simulink model "Model"  (R2015b)
settings: Solver=ode4  StartTime=0.0  StopTime=15  FixedStep=0.015  RelTol=1e-3
undefined symbols (not defined in the file or in its folder): Earth, WGS84
libraries: aerolibutil x3, aerolibfltsims x2, aerolibtransform2 x1
settings Model: Creator=A7med Al-Dakrory  LastModifiedBy=Ahmed
settings DataIOCC: SaveFormat=Array
settings DebuggingCC: AllowSymbolicDim=on
settings HardwareCC: ProdBitPerPointer=32  ProdLargestAtomicFloat=None  ProdIntDivRoundTo=Undefined  ProdEndianess=Unspecified  ProdWordSize=32  ProdHWDeviceType=32-bit Generic
settings GRTTargetCC: GeneratePreprocessorConditionals=Disable all
settings ConfigComp: CovModelRefEnable=Off

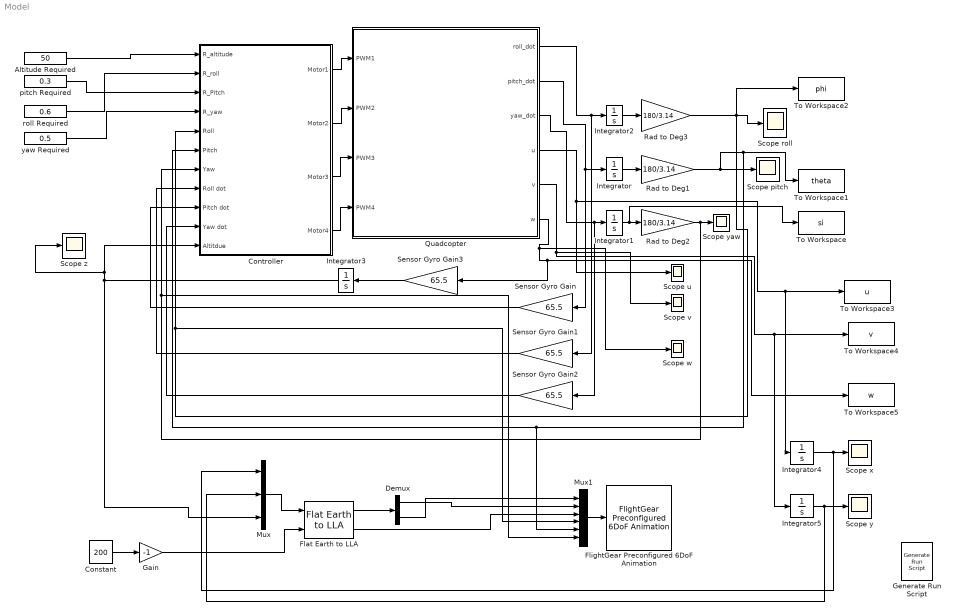
== system Model ==
  Altitude Required : Constant  Value=50
  Constant : Constant  Value=200
  Controller : Subsystem
  Demux : Demux  Outputs=2
  Flat Earth to LLA : aerolibtransform2/Flat Earth to LLA  units=Metric (MKS)  ptype=Earth (WGS84)  F=1/298.257223563  R=6378137  LL0=[34.9100 -117.8912]  psi=0
  FlightGear Preconfigured 6DoF Animation : aerolibfltsims/FlightGear Preconfigured 6DoF Animation  xFlightGearVersion=v3.0  DestinationIpAddress=127.0.0.1  DestinationPort=5502  SampleTime=15/1000
  Gain : Gain  Gain=-1
  Generate Run Script : aerolibfltsims/Generate Run Script  OutputFileName=runfg.bat  FlightGearBaseDirectory=C:\Program Files\FlightGear  GeometryModelName=HL20  DestinationPort=5502  OriginAddress=127.0.0.1  OriginPort=5505  LocalAddress=127.0.0.1  AirportId=KSFO  RunwayId=10L  InitialAltitude=200  InitialHeading=0  OffsetDistance=0  OffsetAzimuth=0  GenerateFile=off  Architecture=Default  dataFlow=Send
  Integrator{,1..5} (6 alike) : Integrator
  Mux : Mux  Inputs=3
  Mux1 : Mux  Inputs=6
  Quadcopter : Subsystem
      mask Display:
      | port_label('output', 1, 'roll_dot')
      | port_label('output', 2, 'pitch_dot')
      | port_label('output', 3, 'yaw_dot')
      | port_label('output', 4, 'u')
      | port_label('output', 5, 'v')
      | port_label('output', 6, 'w')
      | port_label('input', 1, 'Motor1')
      | port_label('input', 2, 'Motor2')
      | port_label('input', 3, 'Motor3')
      | port_label('input', 4, 'Motor4')
  Rad to Deg1 : Gain  Gain=180/3.14
  Rad to Deg2 : Gain  Gain=180/3.14
  Rad to Deg3 : Gain  Gain=180/3.14
  Scope pitch : Scope
  Scope roll : Scope
  Scope u : Scope
  Scope v : Scope
  Scope w : Scope
  Scope x : Scope
  "Scope y " : Scope
  Scope yaw : Scope
  Scope z : Scope
  Sensor Gyro Gain{,1..3} (4 alike) : Gain  Gain=65.5
  To Workspace : ToWorkspace  VariableName=si  SaveFormat=Timeseries  SampleTime=-1
  To Workspace1 : ToWorkspace  VariableName=theta  SaveFormat=Timeseries  SampleTime=-1
  To Workspace2 : ToWorkspace  VariableName=phi  SaveFormat=Timeseries  SampleTime=-1
  To Workspace3 : ToWorkspace  VariableName=u  SaveFormat=Timeseries  SampleTime=-1
  To Workspace4 : ToWorkspace  VariableName=v  SaveFormat=Timeseries  SampleTime=-1
  To Workspace5 : ToWorkspace  VariableName=w  SaveFormat=Timeseries  SampleTime=-1
  pitch Required : Constant  Value=0.3
  roll Required : Constant  Value=0.6
  yaw Required : Constant  Value=0.5
  wires:
  Rad to Deg1/1 -> Mux1/5, Controller/6(Pitch), To Workspace1/1, Scope pitch/1
  Integrator/1 -> Rad to Deg1/1
  Quadcopter/2(pitch_dot) -> Sensor Gyro Gain/1, Integrator/1
  Integrator1/1 -> To Workspace/1, Rad to Deg2/1
  Quadcopter/3(yaw_dot) -> Sensor Gyro Gain2/1, Integrator1/1
  Rad to Deg2/1 -> Controller/7(Yaw), Mux1/6, Scope yaw/1
  Integrator2/1 -> Rad to Deg3/1
  Quadcopter/1(roll_dot) -> Sensor Gyro Gain1/1, Integrator2/1
  Quadcopter/4(u) -> Integrator4/1, To Workspace3/1, Scope u/1
  Quadcopter/5(v) -> Integrator5/1, To Workspace4/1, Scope v/1
  Quadcopter/6(w) -> Sensor Gyro Gain3/1, To Workspace5/1, Scope w/1
  Controller/4(Motor4) -> Quadcopter/4(PWM4)
  Rad to Deg3/1 -> Scope roll/1, To Workspace2/1, Controller/5(Roll), Mux1/4
  Integrator3/1 -> Controller/11(Altitdue), Scope z/1, Mux/3
  Controller/3(Motor3) -> Quadcopter/3(PWM3)
  Controller/2(Motor2) -> Quadcopter/2(PWM2)
  Controller/1(Motor1) -> Quadcopter/1(PWM1)
  Altitude Required/1 -> Controller/1(R_altitude)
  yaw Required/1 -> Controller/4(R_yaw)
  pitch Required/1 -> Controller/3(R_Pitch)
  roll Required/1 -> Controller/2(R_roll)
  Sensor Gyro Gain2/1 -> Controller/10(Yaw dot)
  Sensor Gyro Gain/1 -> Controller/9(Pitch dot)
  Sensor Gyro Gain1/1 -> Controller/8(Roll dot)
  Sensor Gyro Gain3/1 -> Integrator3/1
  Mux/1 -> Flat Earth to LLA/1
  Integrator5/1 -> Mux/2, "Scope y "/1
  Integrator4/1 -> Mux/1, Scope x/1
  Flat Earth to LLA/1 -> Demux/1
  Mux1/1 -> FlightGear Preconfigured 6DoF Animation/1
  Flat Earth to LLA/2 -> Mux1/3
  Gain/1 -> Flat Earth to LLA/2
  Demux/1 -> Mux1/2
  Demux/2 -> Mux1/1
  Constant/1 -> Gain/1

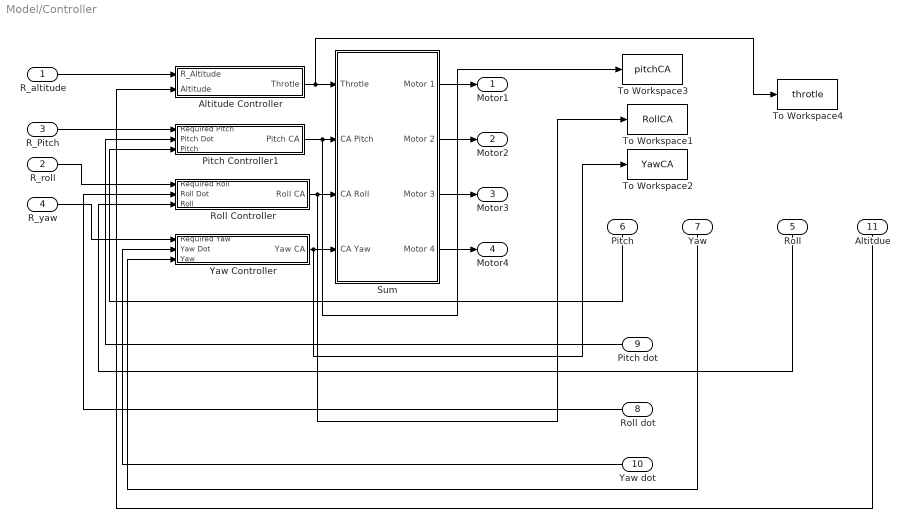
== system Model/Controller ==
  R_altitude : Inport
  R_roll : Inport  Port=2
  R_Pitch : Inport  Port=3
  R_yaw : Inport  Port=4
  Roll : Inport  Port=5
  Pitch : Inport  Port=6
  Yaw : Inport  Port=7
  Roll dot : Inport  Port=8
  Pitch dot : Inport  Port=9
  Yaw dot : Inport  Port=10
  Altitdue : Inport  Port=11
  Altitude Controller : Subsystem
  Pitch Controller1 : Subsystem
  Roll Controller : Subsystem
  Sum : Subsystem
  To Workspace1 : ToWorkspace  VariableName=RollCA  SaveFormat=Timeseries  SampleTime=-1
  To Workspace2 : ToWorkspace  VariableName=YawCA  SaveFormat=Timeseries  SampleTime=-1
  To Workspace3 : ToWorkspace  VariableName=pitchCA  SaveFormat=Timeseries  SampleTime=-1
  To Workspace4 : ToWorkspace  VariableName=throtle  SaveFormat=Timeseries  SampleTime=-1
  Yaw Controller : Subsystem
  Motor1 : Outport
  Motor2 : Outport  Port=2
  Motor3 : Outport  Port=3
  Motor4 : Outport  Port=4
  wires:
  Pitch Controller1/1(Pitch CA) -> To Workspace3/1, Sum/2(CA Pitch)
  Pitch dot/1 -> Pitch Controller1/2(Pitch Dot)
  R_Pitch/1 -> Pitch Controller1/1(Required Pitch)
  Sum/1(Motor 1) -> Motor1/1
  Sum/2(Motor 2) -> Motor2/1
  Sum/3(Motor 3) -> Motor3/1
  Sum/4(Motor 4) -> Motor4/1
  Roll dot/1 -> Roll Controller/2(Roll Dot)
  Yaw/1 -> Yaw Controller/3(Yaw)
  Roll/1 -> Roll Controller/3(Roll)
  Pitch/1 -> Pitch Controller1/3(Pitch)
  Yaw dot/1 -> Yaw Controller/2(Yaw Dot)
  Roll Controller/1(Roll CA) -> To Workspace1/1, Sum/3(CA Roll)
  Yaw Controller/1(Yaw CA) -> To Workspace2/1, Sum/4(CA Yaw)
  R_roll/1 -> Roll Controller/1(Required Roll)
  R_yaw/1 -> Yaw Controller/1(Required Yaw)
  R_altitude/1 -> Altitude Controller/1(R_Altitude)
  Altitude Controller/1(Throtle) -> To Workspace4/1, Sum/1(Throtle)
  Altitdue/1 -> Altitude Controller/2(Altitude)

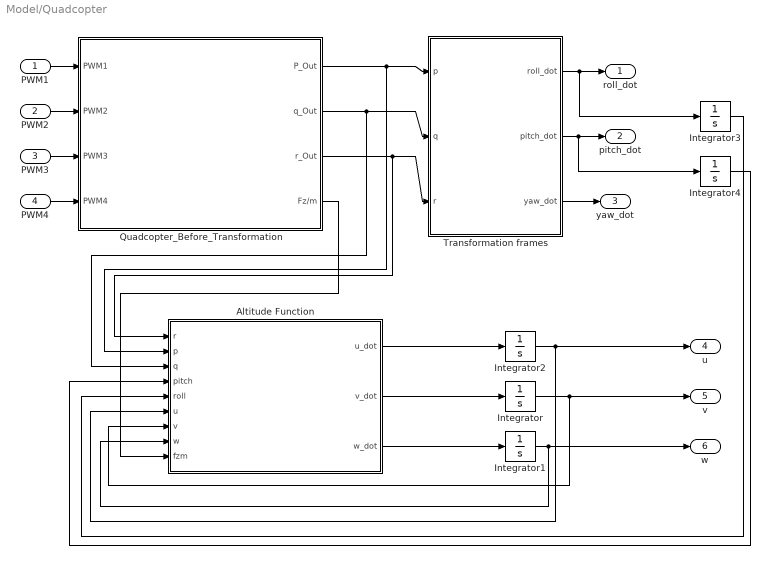
== system Model/Quadcopter ==
  PWM1 : Inport
  PWM2 : Inport  Port=2
  PWM3 : Inport  Port=3
  PWM4 : Inport  Port=4
  Altitude Function : MATLAB Function  TreatAsAtomicUnit=on
      settings: PermitHierarchicalResolution=ParametersOnly
  Integrator{,1..4} (5 alike) : Integrator
  Quadcopter_Before_Transformation : Subsystem
      mask Display:
      | port_label('output', 1, 'roll rate')
      | port_label('output', 2, 'pitch rate')
      | port_label('output', 3, 'yaw rate')
      | port_label('output', 4, 'Fz/m')
      | port_label('input', 1, 'PWM 1')
      | port_label('input', 2, 'PWM 2')
      | port_label('input', 3, 'PWM 3')
      | port_label('input', 4, 'PWM 4')
  Transformation frames : Subsystem
  roll_dot : Outport
  pitch_dot : Outport  Port=2
  yaw_dot : Outport  Port=3
  u : Outport  Port=4
  v : Outport  Port=5
  w : Outport  Port=6
  wires:
  PWM2/1 -> Quadcopter_Before_Transformation/2(PWM2)
  Quadcopter_Before_Transformation/3(r_Out) -> Altitude Function/1(r), Transformation frames/3(r)
  Quadcopter_Before_Transformation/1(P_Out) -> Altitude Function/2(p), Transformation frames/1(p)
  PWM1/1 -> Quadcopter_Before_Transformation/1(PWM1)
  Quadcopter_Before_Transformation/2(q_Out) -> Altitude Function/3(q), Transformation frames/2(q)
  Transformation frames/2(pitch_dot) -> Integrator4/1, pitch_dot/1
  Transformation frames/3(yaw_dot) -> yaw_dot/1
  Transformation frames/1(roll_dot) -> Integrator3/1, roll_dot/1
  PWM3/1 -> Quadcopter_Before_Transformation/3(PWM3)
  PWM4/1 -> Quadcopter_Before_Transformation/4(PWM4)
  Altitude Function/2(v_dot) -> Integrator/1
  Altitude Function/3(w_dot) -> Integrator1/1
  Altitude Function/1(u_dot) -> Integrator2/1
  Integrator4/1 -> Altitude Function/4(pitch)
  Integrator3/1 -> Altitude Function/5(roll)
  Integrator2/1 -> u/1, Altitude Function/6(u)
  Integrator/1 -> Altitude Function/7(v), v/1
  Integrator1/1 -> Altitude Function/8(w), w/1
  Quadcopter_Before_Transformation/4(Fz/m) -> Altitude Function/9(fzm)

== system Model/Controller/Altitude Controller ==
  R_Altitude : Inport
  Altitude : Inport  Port=2
  PID Altitude : Subsystem
  Sum : Sum  Inputs=|+-
  Throtle : Outport
  wires:
  Sum/1 -> PID Altitude/1(Error)
  R_Altitude/1 -> Sum/2
  Altitude/1 -> Sum/1
  PID Altitude/1(Output) -> Throtle/1

== system Model/Controller/Pitch Controller1 ==
  Required Pitch : Inport
  Pitch Dot : Inport  Port=2
  Pitch : Inport  Port=3
  PID Pitch : Subsystem
  PID Pitch Rate : Subsystem
  Sum2 : Sum  Inputs=|++
  Sum3 : Sum  Inputs=|+-
  Pitch CA : Outport
  wires:
  Required Pitch/1 -> Sum3/1
  Sum3/1 -> PID Pitch/1(Error)
  Pitch Dot/1 -> PID Pitch Rate/1(Error)
  Pitch/1 -> Sum3/2
  PID Pitch/1(Output) -> Sum2/1
  PID Pitch Rate/1(Output) -> Sum2/2
  Sum2/1 -> Pitch CA/1

== system Model/Controller/Roll Controller ==
  Required Roll : Inport
  Roll Dot : Inport  Port=2
  Roll : Inport  Port=3
  PID Roll : Subsystem
  PID Roll Rate : Subsystem
  Sum2 : Sum  Inputs=|++
  Sum3 : Sum  Inputs=|+-
  Roll CA : Outport
  wires:
  Required Roll/1 -> Sum3/1
  Sum3/1 -> PID Roll/1(Error)
  Roll Dot/1 -> PID Roll Rate/1(Error)
  Roll/1 -> Sum3/2
  PID Roll/1(Output) -> Sum2/1
  PID Roll Rate/1(Output) -> Sum2/2
  Sum2/1 -> Roll CA/1

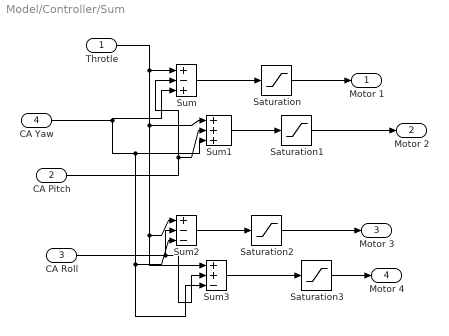
== system Model/Controller/Sum ==
  Throtle : Inport
  CA Pitch : Inport  Port=2
  CA Roll : Inport  Port=3
  CA Yaw : Inport  Port=4
  Saturation{,1..3} (4 alike) : Saturate  UpperLimit=1950  LowerLimit=1050
  Sum : Sum  Inputs=+-+
  Sum1 : Sum  Inputs=+++
  Sum2 : Sum  Inputs=+--
  Sum3 : Sum  Inputs=++-
  Motor 1 : Outport
  Motor 2 : Outport  Port=2
  Motor 3 : Outport  Port=3
  Motor 4 : Outport  Port=4
  wires:
  CA Pitch/1 -> Sum/2, Sum1/2
  Saturation/1 -> Motor 1/1
  Sum/1 -> Saturation/1
  Sum1/1 -> Saturation1/1
  Saturation1/1 -> Motor 2/1
  Throtle/1 -> Sum3/1, Sum2/1, Sum1/1, Sum/1
  CA Roll/1 -> Sum3/2, Sum2/2
  Saturation2/1 -> Motor 3/1
  Sum2/1 -> Saturation2/1
  Sum3/1 -> Saturation3/1
  Saturation3/1 -> Motor 4/1
  CA Yaw/1 -> Sum/3, Sum3/3, Sum2/3, Sum1/3

== system Model/Controller/Yaw Controller ==
  Required Yaw : Inport
  Yaw Dot : Inport  Port=2
  Yaw : Inport  Port=3
  PID Yaw : Subsystem
  PID Yaw Rate : Subsystem
  Sum2 : Sum  Inputs=|++
  Sum3 : Sum  Inputs=|+-
  Yaw CA : Outport
  wires:
  Required Yaw/1 -> Sum3/1
  Sum3/1 -> PID Yaw/1(Error)
  Yaw Dot/1 -> PID Yaw Rate/1(Error)
  Yaw/1 -> Sum3/2
  PID Yaw/1(Output) -> Sum2/1
  PID Yaw Rate/1(Output) -> Sum2/2
  Sum2/1 -> Yaw CA/1

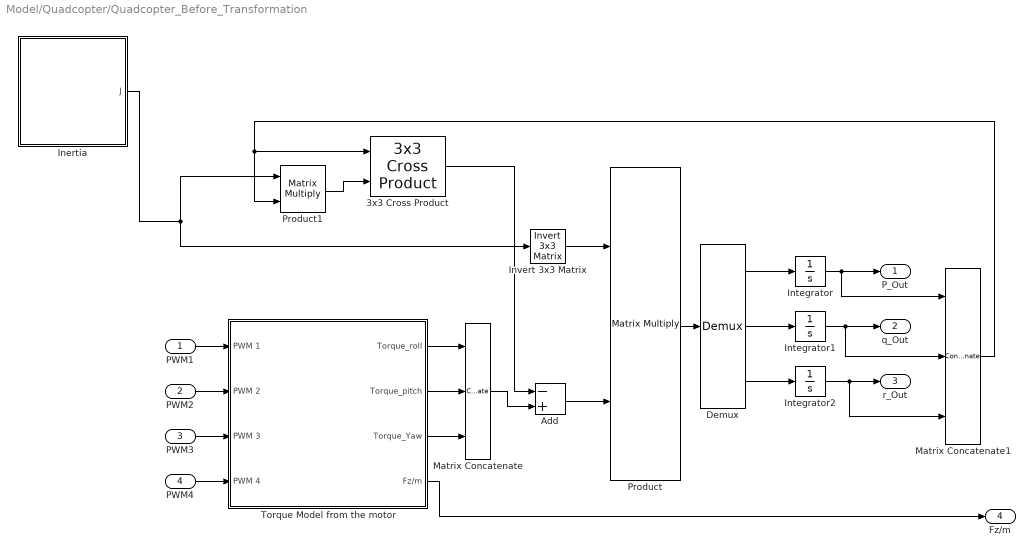
== system Model/Quadcopter/Quadcopter_Before_Transformation ==
  PWM1 : Inport
  PWM2 : Inport  Port=2
  PWM3 : Inport  Port=3
  PWM4 : Inport  Port=4
  3x3 Cross Product : aerolibutil/3x3 Cross Product
  Add : Sum  Inputs=-+
  Demux : Demux  Outputs=3
  Inertia : Subsystem
  Integrator : Integrator
  Integrator1 : Integrator
  Integrator2 : Integrator
  Invert 3x3 Matrix : aerolibutil/Invert  3x3 Matrix
  Matrix Concatenate : Concatenate  NumInputs=3  ConcatenateDimension=2
  Matrix Concatenate1 : Concatenate  NumInputs=3  ConcatenateDimension=2
  Product : Product  Multiplication=Matrix(*)
  Product1 : Product  Multiplication=Matrix(*)
  Torque Model from the motor : Subsystem
      mask Display:
      | port_label('output', 1, 'Torque_Roll')
      | port_label('output', 2, 'Torque_pitch')
      | port_label('output', 3, 'Torque_yaw')
      | port_label('output', 4, 'Fz/m')
      | port_label('input', 1, 'PWM 1')
      | port_label('input', 2, 'PWM 2')
      | port_label('input', 3, 'PWM 3')
      | port_label('input', 4, 'PWM 4')
  P_Out : Outport
  q_Out : Outport  Port=2
  r_Out : Outport  Port=3
  Fz/m : Outport  Port=4
  wires:
  Demux/1 -> Integrator/1
  Torque Model from the motor/1("Torque_roll ") -> Matrix Concatenate/1
  Product/1 -> Demux/1
  Integrator2/1 -> Matrix Concatenate1/3, r_Out/1
  Integrator/1 -> Matrix Concatenate1/1, P_Out/1
  Integrator1/1 -> Matrix Concatenate1/2, q_Out/1
  PWM2/1 -> Torque Model from the motor/2(PWM 2)
  PWM4/1 -> Torque Model from the motor/4(PWM 4)
  PWM3/1 -> Torque Model from the motor/3(PWM 3)
  PWM1/1 -> Torque Model from the motor/1(PWM 1)
  Invert 3x3 Matrix/1 -> Product/1
  Demux/3 -> Integrator2/1
  Demux/2 -> Integrator1/1
  Torque Model from the motor/2(Torque_pitch) -> Matrix Concatenate/2
  Torque Model from the motor/3("Torque_Yaw ") -> Matrix Concatenate/3
  Matrix Concatenate/1 -> Add/2
  Add/1 -> Product/2
  Matrix Concatenate1/1 -> Product1/2, 3x3 Cross Product/1
  Inertia/1(J) -> Invert 3x3 Matrix/1, Product1/1
  Product1/1 -> 3x3 Cross Product/2
  3x3 Cross Product/1 -> Add/1
  Torque Model from the motor/4(Fz/m) -> Fz/m/1

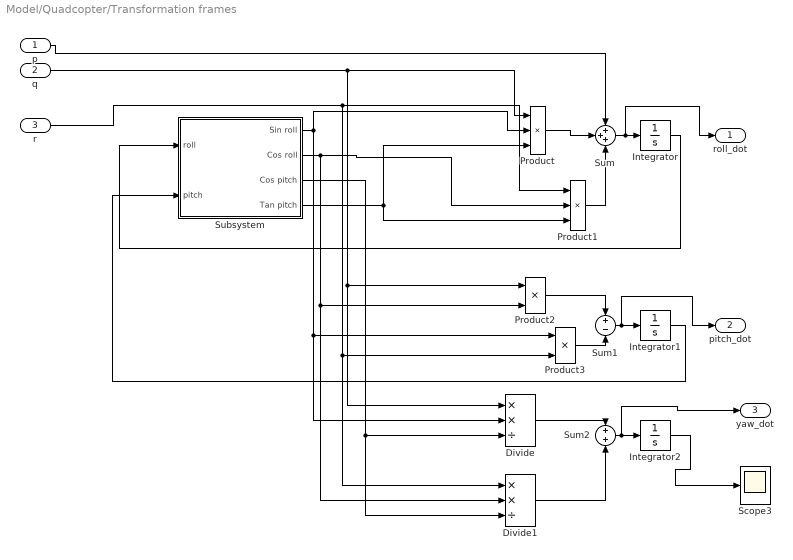
== system Model/Quadcopter/Transformation frames ==
  p : Inport
  q : Inport  Port=2
  r : Inport  Port=3
  Divide : Product  Inputs=**/
  Divide1 : Product  Inputs=**/
  Integrator : Integrator
  Integrator1 : Integrator
  Integrator2 : Integrator
  Product : Product  Inputs=3
  Product1 : Product  Inputs=3
  Product2 : Product
  Product3 : Product
  Scope3 : Scope
  Subsystem : Subsystem
  Sum : Sum  Inputs=+++
  Sum1 : Sum  Inputs=+-
  Sum2 : Sum
  roll_dot : Outport
  pitch_dot : Outport  Port=2
  yaw_dot : Outport  Port=3
  wires:
  Integrator/1 -> Subsystem/1(roll)
  p/1 -> Sum/1
  Subsystem/2(Cos roll) -> Divide1/2, Product2/2, Product1/2
  Sum/1 -> roll_dot/1, Integrator/1
  Subsystem/4(Tan pitch) -> Product1/3, Product/3
  q/1 -> Divide/1, Product2/1, Product/1
  r/1 -> Divide1/1, Product3/2, Product1/1
  Sum2/1 -> yaw_dot/1, Integrator2/1
  Sum1/1 -> pitch_dot/1, Integrator1/1
  Integrator1/1 -> Subsystem/2(pitch)
  Subsystem/1(Sin roll) -> Divide/2, Product3/1, Product/2
  Integrator2/1 -> Scope3/1
  Product/1 -> Sum/2
  Product1/1 -> Sum/3
  Product2/1 -> Sum1/1
  Product3/1 -> Sum1/2
  Divide/1 -> Sum2/1
  Subsystem/3(Cos pitch) -> Divide1/3, Divide/3
  Divide1/1 -> Sum2/2

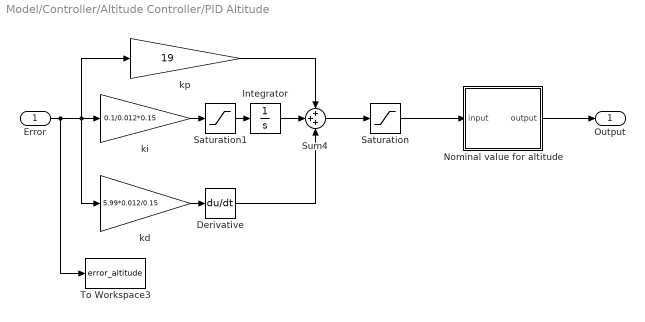
== system Model/Controller/Altitude Controller/PID Altitude ==
  Error : Inport
  Derivative : Derivative
  Integrator : Integrator
  Nominal value for altitude : MATLAB Function  TreatAsAtomicUnit=on
      settings: PermitHierarchicalResolution=ParametersOnly
  Saturation : Saturate  UpperLimit=20  LowerLimit=0
  Saturation1 : Saturate  UpperLimit=20  LowerLimit=-20
  Sum4 : Sum  Inputs=+++
  To Workspace3 : ToWorkspace  VariableName=error_altitude  SaveFormat=Timeseries  SampleTime=-1
  kd : Gain  Gain=5.99*0.012/0.15
  ki : Gain  Gain=0.1/0.012*0.15
  kp : Gain  Gain=19
  Output : Outport
  wires:
  Integrator/1 -> Sum4/2
  kd/1 -> Derivative/1
  Error/1 -> To Workspace3/1, kd/1, ki/1, kp/1
  kp/1 -> Sum4/1
  Derivative/1 -> Sum4/3
  Sum4/1 -> Saturation/1
  Saturation/1 -> Nominal value for altitude/1(input)
  Nominal value for altitude/1(output) -> Output/1
  ki/1 -> Saturation1/1
  Saturation1/1 -> Integrator/1

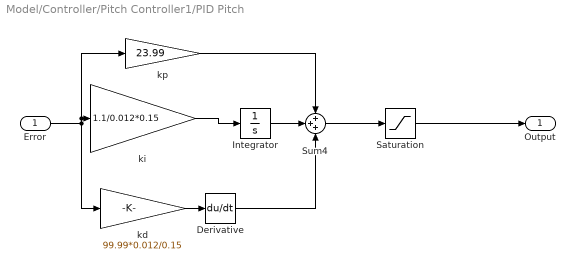
== system Model/Controller/Pitch Controller1/PID Pitch ==
  Error : Inport
  Derivative : Derivative
  Integrator : Integrator
  Saturation : Saturate  UpperLimit=150  LowerLimit=-150
  Sum4 : Sum  Inputs=+++
  kd : Gain  Gain=99.99*0.012/0.15
  ki : Gain  Gain=1.1/0.012*0.15
  kp : Gain  Gain=23.99
  Output : Outport
  wires:
  Integrator/1 -> Sum4/2
  kd/1 -> Derivative/1
  Error/1 -> ki/1, kp/1, kd/1
  kp/1 -> Sum4/1
  Derivative/1 -> Sum4/3
  ki/1 -> Integrator/1
  Saturation/1 -> Output/1
  Sum4/1 -> Saturation/1

== system Model/Controller/Pitch Controller1/PID Pitch Rate ==
  Error : Inport
  Derivative : Derivative
  Integrator : Integrator
  Sum4 : Sum  Inputs=+++
  kd : Gain  Gain=-89.99*0.01*0.012/0.15
  ki : Gain  Gain=0
  kp : Gain  Gain=-0.01*23.9
  Output : Outport
  wires:
  ki/1 -> Integrator/1
  Derivative/1 -> Sum4/3
  kp/1 -> Sum4/1
  Error/1 -> kd/1, kp/1, ki/1
  kd/1 -> Derivative/1
  Integrator/1 -> Sum4/2
  Sum4/1 -> Output/1

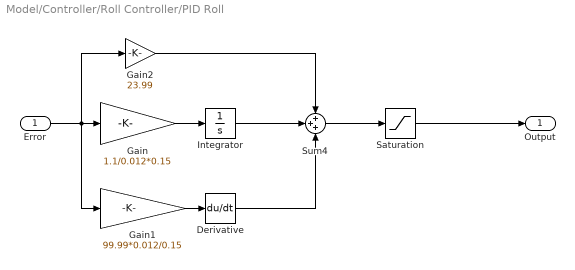
== system Model/Controller/Roll Controller/PID Roll ==
  Error : Inport
  Derivative : Derivative
  Gain : Gain  Gain=1.1/0.012*0.15
  Gain1 : Gain  Gain=99.99*0.012/0.15
  Gain2 : Gain  Gain=23.99
  Integrator : Integrator
  Saturation : Saturate  UpperLimit=150  LowerLimit=-150
  Sum4 : Sum  Inputs=+++
  Output : Outport
  wires:
  Integrator/1 -> Sum4/2
  Gain1/1 -> Derivative/1
  Error/1 -> Gain1/1, Gain/1, Gain2/1
  Gain2/1 -> Sum4/1
  Derivative/1 -> Sum4/3
  Gain/1 -> Integrator/1
  Saturation/1 -> Output/1
  Sum4/1 -> Saturation/1

== system Model/Controller/Roll Controller/PID Roll Rate ==
  Error : Inport
  Derivative : Derivative
  Gain : Gain  Gain=0
  Gain1 : Gain  Gain=-89.99*0.01*0.012/0.15
  Gain2 : Gain  Gain=-0.01*23.9
  Integrator : Integrator
  Sum4 : Sum  Inputs=+++
  Output : Outport
  wires:
  Gain/1 -> Integrator/1
  Derivative/1 -> Sum4/3
  Gain2/1 -> Sum4/1
  Error/1 -> Gain1/1, Gain2/1, Gain/1
  Gain1/1 -> Derivative/1
  Integrator/1 -> Sum4/2
  Sum4/1 -> Output/1

== system Model/Controller/Yaw Controller/PID Yaw ==
  Error : Inport
  Derivative : Derivative
  Gain : Gain  Gain=1.1/0.012*0.15
  Gain1 : Gain  Gain=99.99*0.012/0.15
  Gain2 : Gain  Gain=23.99
  Integrator : Integrator
  Saturation : Saturate  UpperLimit=150  LowerLimit=-150
  Sum4 : Sum  Inputs=+++
  Output : Outport
  wires:
  Integrator/1 -> Sum4/2
  Gain1/1 -> Derivative/1
  Error/1 -> Gain1/1, Gain/1, Gain2/1
  Gain2/1 -> Sum4/1
  Derivative/1 -> Sum4/3
  Gain/1 -> Integrator/1
  Saturation/1 -> Output/1
  Sum4/1 -> Saturation/1

== system Model/Controller/Yaw Controller/PID Yaw Rate ==
  Error : Inport
  Derivative : Derivative
  Gain : Gain  Gain=0
  Gain1 : Gain  Gain=-89.99*0.01*0.012/0.15
  Gain2 : Gain  Gain=-0.01*23.9
  Integrator : Integrator
  Sum4 : Sum  Inputs=+++
  Output : Outport
  wires:
  Gain/1 -> Integrator/1
  Derivative/1 -> Sum4/3
  Gain2/1 -> Sum4/1
  Error/1 -> Gain1/1, Gain2/1, Gain/1
  Gain1/1 -> Derivative/1
  Integrator/1 -> Sum4/2
  Sum4/1 -> Output/1

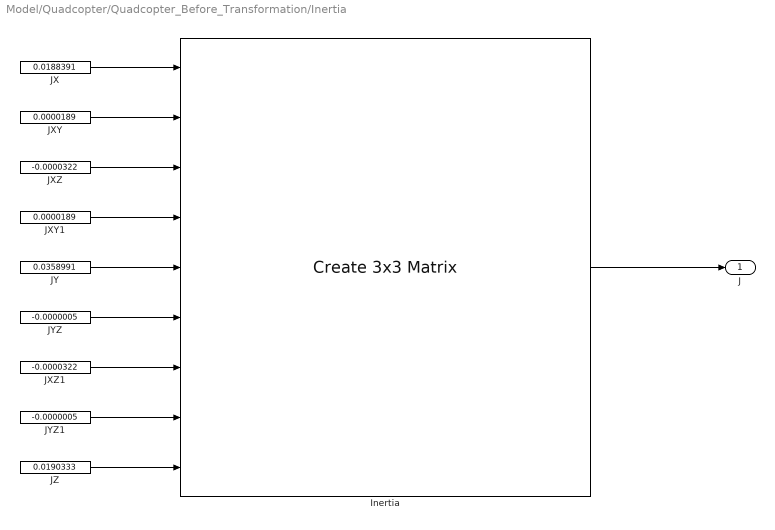
== system Model/Quadcopter/Quadcopter_Before_Transformation/Inertia ==
  Inertia : aerolibutil/Create 3x3 Matrix
  JX : Constant  Value=0.0188391
  JXY : Constant  Value=0.0000189
  JXY1 : Constant  Value=0.0000189
  JXZ : Constant  Value=-0.0000322
  JXZ1 : Constant  Value=-0.0000322
  JY : Constant  Value=0.0358991
  JYZ : Constant  Value=-0.0000005
  JYZ1 : Constant  Value=-0.0000005
  JZ : Constant  Value=0.0190333
  J : Outport
  wires:
  JYZ/1 -> Inertia/6
  JZ/1 -> Inertia/9
  JXY/1 -> Inertia/2
  JXZ/1 -> Inertia/3
  JY/1 -> Inertia/5
  JX/1 -> Inertia/1
  Inertia/1 -> J/1
  JXY1/1 -> Inertia/4
  JXZ1/1 -> Inertia/7
  JYZ1/1 -> Inertia/8

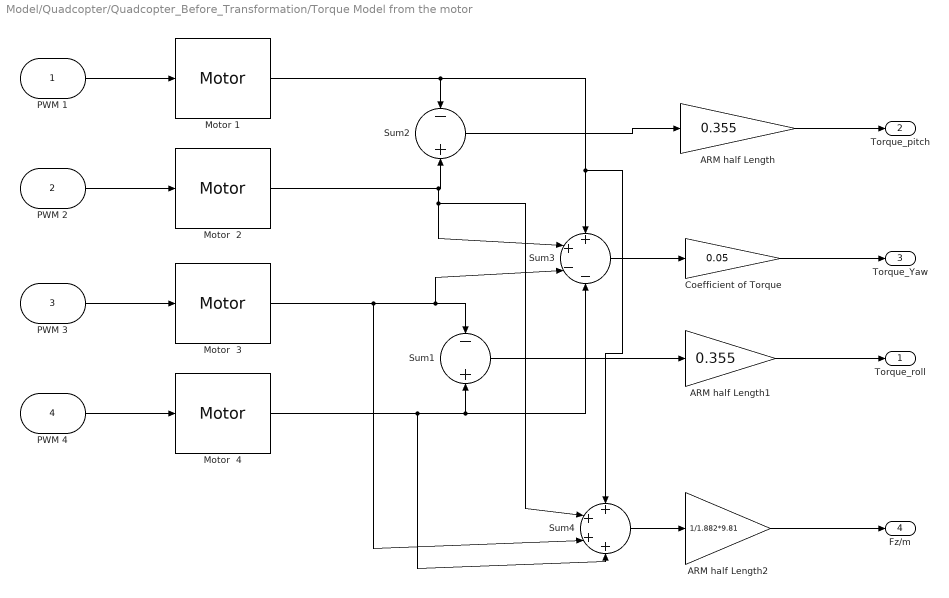
== system Model/Quadcopter/Quadcopter_Before_Transformation/Torque Model from the motor ==
  PWM 1 : Inport
  PWM 2 : Inport  Port=2
  PWM 3 : Inport  Port=3
  PWM 4 : Inport  Port=4
  ARM half Length : Gain  Gain=0.355
  ARM half Length1 : Gain  Gain=0.355
  ARM half Length2 : Gain  Gain=1/1.882*9.81
  Coefficient of Torque : Gain  Gain=0.05
  Motor  2 : MATLABFcn  MATLABFcn=Motor
  Motor  3 : MATLABFcn  MATLABFcn=Motor
  Motor  4 : MATLABFcn  MATLABFcn=Motor
  Motor 1 : MATLABFcn  MATLABFcn=Motor
  Sum1 : Sum  Inputs=-+
  Sum2 : Sum  Inputs=-+
  Sum3 : Sum  Inputs=++--
  Sum4 : Sum  Inputs=++++
  "Torque_roll " : Outport
  Torque_pitch : Outport  Port=2
  "Torque_Yaw " : Outport  Port=3
  Fz/m : Outport  Port=4
  wires:
  Sum3/1 -> Coefficient of Torque/1
  Sum1/1 -> ARM half Length1/1
  Sum2/1 -> ARM half Length/1
  ARM half Length/1 -> Torque_pitch/1
  PWM 1/1 -> Motor 1/1
  PWM 2/1 -> Motor  2/1
  PWM 3/1 -> Motor  3/1
  PWM 4/1 -> Motor  4/1
  ARM half Length1/1 -> "Torque_roll "/1
  Coefficient of Torque/1 -> "Torque_Yaw "/1
  Motor 1/1 -> Sum4/1, Sum3/1, Sum2/1
  Motor  2/1 -> Sum4/2, Sum3/2, Sum2/2
  Motor  3/1 -> Sum4/3, Sum3/3, Sum1/1
  Motor  4/1 -> Sum4/4, Sum3/4, Sum1/2
  Sum4/1 -> ARM half Length2/1
  ARM half Length2/1 -> Fz/m/1

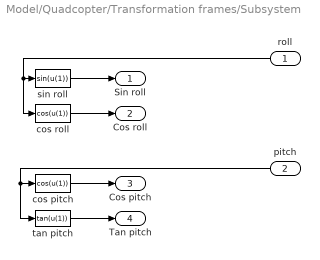
== system Model/Quadcopter/Transformation frames/Subsystem ==
  roll : Inport
  pitch : Inport  Port=2
  cos pitch : Fcn  Expr=cos(u(1))
  cos roll : Fcn  Expr=cos(u(1))
  sin roll : Fcn  Expr=sin(u(1))
  tan pitch : Fcn  Expr=tan(u(1))
  Sin roll : Outport
  Cos roll : Outport  Port=2
  Cos pitch : Outport  Port=3
  Tan pitch : Outport  Port=4
  wires:
  roll/1 -> sin roll/1, cos roll/1
  cos pitch/1 -> Cos pitch/1
  sin roll/1 -> Sin roll/1
  tan pitch/1 -> Tan pitch/1
  cos roll/1 -> Cos roll/1
  pitch/1 -> cos pitch/1, tan pitch/1

== matlab function Model/Quadcopter/Altitude Function ==
  data: r input; p input; q input; pitch input; roll input; u input; u_dot output; v input; w input; fzm input; v_dot output; w_dot output
function [u_dot,v_dot,w_dot] = fcn(r,p,q,pitch,roll,u,v,w,fzm)
%#codegen
u_dot=(r*v-q*w)-9.81*sin(pitch)+0;
v_dot=(p*w-r*u)+9.81*cos(pitch)*sin(roll)+0;
w_dot=(q*u-p*v)+9.81*cos(pitch)*cos(roll)-fzm;

== matlab function Model/Controller/Altitude Controller/PID Altitude/Nominal value for altitude ==
  data: input input; output output
function output  = fcn(input)

output=1000+33*input;
